simulink model "RotationalPendulum_Linear_2021b"  (R2025b)
settings: Solver=VariableStepAuto
libraries: cstblocks x1
settings Model: Creator=djangovanderplas  LastModifiedBy=thoma

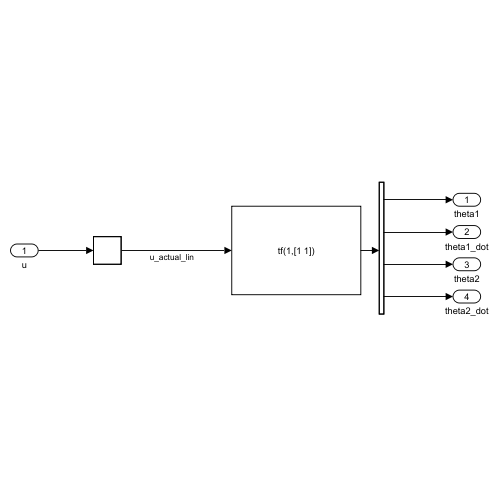
[thumbnail: Simulink's stored preview of the top-level diagram]
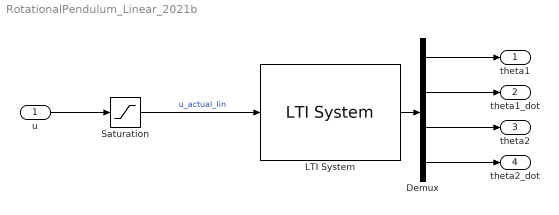
== system RotationalPendulum_Linear_2021b ==
  u : Inport
  Demux : Demux
  LTI System : cstblocks/LTI System  sys=linsys1  IC=x0  PadeOrder=0
  Saturation : Saturate  UpperLimit=1  LowerLimit=-1
  theta1 : Outport
  theta1_dot : Outport  Port=2
  theta2 : Outport  Port=3
  theta2_dot : Outport  Port=4
  wires:
  u/1 -> Saturation/1
  LTI System/1 -> Demux/1
  Demux/1 -> theta1/1
  Demux/2 -> theta1_dot/1
  Demux/3 -> theta2/1
  Demux/4 -> theta2_dot/1
  Saturation/1 -> LTI System/1  "u_actual_lin"
